simulink model "controllabexpt1n2"  (R2023b)
settings: Solver=VariableStepAuto  StartTime=0.0  StopTime=200  RelTol=1e-3
settings Model: Creator=hp  LastModifiedBy=LABA

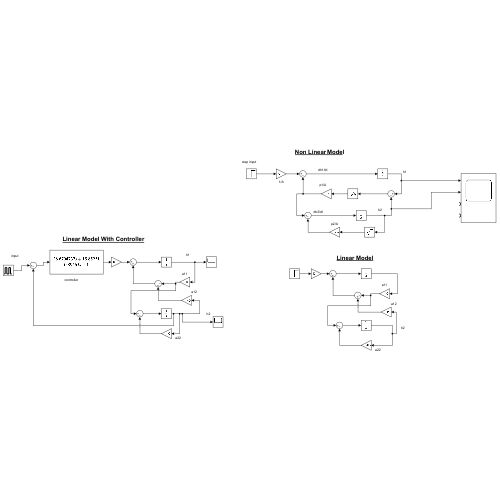
[thumbnail: Simulink's stored preview of the top-level diagram]
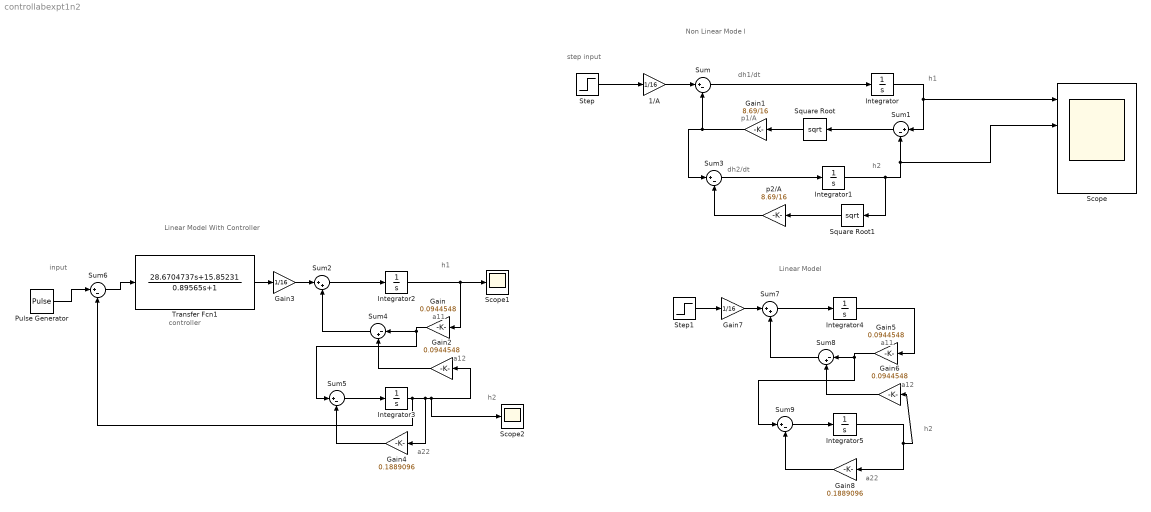
== system controllabexpt1n2 ==
  note: Linear Model With Controller
  note: h1
  note: Linear Model
  note: Non Linear Mode l
  note: h2
  note: controller
  note: input
  note: a22
  note: a12
  note: a11
  note: step input
  note: p1/A
  note: dh2/dt
  note: dh1/dt
  note: h2
  note: h1
  note: h2
  note: a12
  note: a22
  note: a11
  1/A : Gain  Gain=1/16
  Gain{,2,5..6} (4 alike) : Gain  Gain=0.0944548
  Gain1 : Gain  Gain=8.69/16
  Gain3 : Gain  Gain=1/16
  Gain4 : Gain  Gain=0.1889096
  Gain7 : Gain  Gain=1/16
  Gain8 : Gain  Gain=0.1889096
  Integrator : Integrator  InitialCondition=15
  Integrator1 : Integrator  InitialCondition=10
  Integrator2 : Integrator  InitialCondition=15
  Integrator3 : Integrator  InitialCondition=10
  Integrator4 : Integrator  InitialCondition=15
  Integrator5 : Integrator  InitialCondition=10
  Pulse Generator : DiscretePulseGenerator  PulseType=Time based  Amplitude=25  Period=70  PulseWidth=50
  Scope : Scope  NumInputPorts=4
  Scope1 : Scope
  Scope2 : Scope
  Square Root : Sqrt
  Square Root1 : Sqrt
  Step : Step  Time=0  After=25  SampleTime=0
  Step1 : Step  After=25  SampleTime=0
  Sum{,1,3,5..6,9} (6 alike) : Sum  Inputs=|+-
  Sum2 : Sum  Inputs=|++
  Sum4 : Sum  Inputs=|-+
  Sum7 : Sum  Inputs=|++
  Sum8 : Sum  Inputs=|-+
  Transfer Fcn1 : TransferFcn  Numerator=[28.6704737 15.85231]  Denominator=[0.89565 1]
  p2/A : Gain  Gain=8.69/16
  wires:
  1/A/1 -> Sum/1
  Gain1/1 -> Sum3/1, Sum/2
  Sum/1 -> Integrator/1
  Sum1/1 -> Square Root/1
  Square Root/1 -> Gain1/1
  p2/A/1 -> Sum3/2
  Sum3/1 -> Integrator1/1
  Square Root1/1 -> p2/A/1
  Step/1 -> 1/A/1
  Integrator/1 -> Sum1/1, Scope/1
  Integrator1/1 -> Sum1/2, Scope/2, Square Root1/1
  Integrator2/1 -> Scope1/1, Gain/1
  Sum2/1 -> Integrator2/1
  Gain/1 -> Sum5/1, Sum4/1
  Gain2/1 -> Sum4/2
  Sum4/1 -> Sum2/2
  Gain3/1 -> Sum2/1
  Sum5/1 -> Integrator3/1
  Gain4/1 -> Sum5/2
  Integrator3/1 -> Scope2/1, Gain2/1, Gain4/1, Sum6/2
  Pulse Generator/1 -> Sum6/1
  Sum6/1 -> Transfer Fcn1/1
  Transfer Fcn1/1 -> Gain3/1
  Step1/1 -> Gain7/1
  Sum7/1 -> Integrator4/1
  Integrator5/1 -> Gain8/1, Gain6/1
  Sum9/1 -> Integrator5/1
  Gain5/1 -> Sum9/1, Sum8/1
  Sum8/1 -> Sum7/2
  Gain7/1 -> Sum7/1
  Gain8/1 -> Sum9/2
  Integrator4/1 -> Gain5/1
  Gain6/1 -> Sum8/2
